simulink model "EMG_Model_Simulink"  (R2019a)
settings: Solver=VariableStepAuto  StartTime=0.0  StopTime=180  RelTol=1e-3
libraries: dsparch4 x2, simulink x1
settings Model: Creator=patri  LastModifiedBy=patri

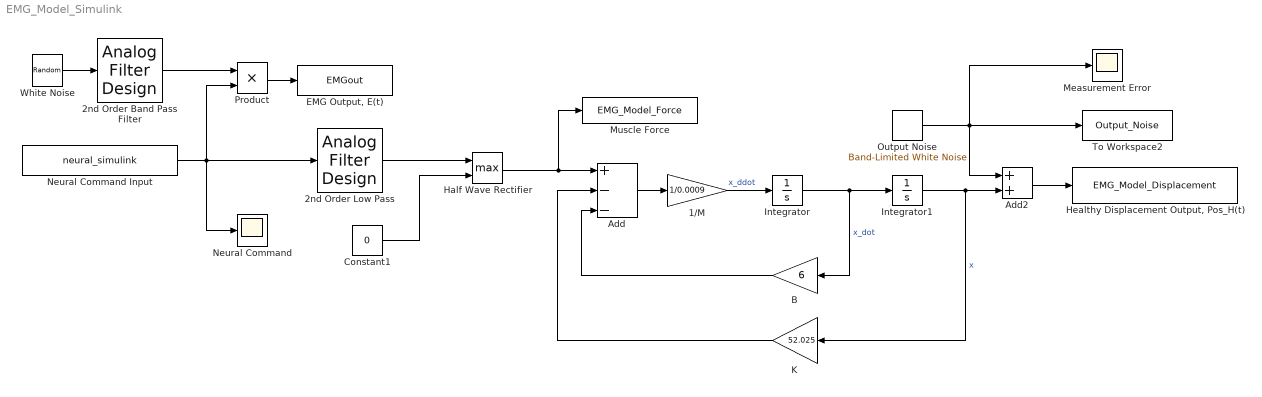
== system EMG_Model_Simulink ==
  1/M : Gain  Gain=1/0.0009
  2nd Order Band Pass Filter : dsparch4/Analog Filter Design  method=Butterworth  filttype=Bandpass  N=2  Wlo=62.83  Whi=3141.59  Rp=2  Rs=40
  2nd Order Low Pass : dsparch4/Analog Filter Design  method=Butterworth  filttype=Lowpass  N=2  Wlo=6.28*2  Whi=80  Rp=2  Rs=40
  Add : Sum  Inputs=+--
  Add2 : Sum
  B : Gain  Gain=6
  Constant1 : Constant  Value=0
  "EMG Output, E(t)" : ToWorkspace  VariableName=EMGout  SampleTime=0.001
  Half Wave Rectifier : MinMax  Function=max  Inputs=2
  "Healthy Displacement Output, Pos_H(t)" : ToWorkspace  VariableName=EMG_Model_Displacement  SampleTime=0.001
  Integrator : Integrator
  Integrator1 : Integrator
  K : Gain  Gain=52.025
  Measurement Error : Scope
  Muscle Force : ToWorkspace  VariableName=EMG_Model_Force  SampleTime=0.001
  Neural Command : Scope
  Neural Command Input : FromWorkspace  VariableName=neural_simulink  SampleTime=0.001
  Output Noise : simulink/Sources/Band-Limited White Noise  Cov=set_output_noise_power  Ts=0.001  seed=22334
  Product : Product
  To Workspace2 : ToWorkspace  VariableName=Output_Noise  SampleTime=0.001
  White Noise : UniformRandomNumber  Minimum=-6.2e-4  Maximum=6.2e-4  SampleTime=0.001
  wires:
  White Noise/1 -> 2nd Order Band Pass Filter/1
  Neural Command Input/1 -> Neural Command/1, 2nd Order Low Pass/1, Product/2
  Add/1 -> 1/M/1
  1/M/1 -> Integrator/1  "x_ddot"
  Integrator/1 -> B/1, Integrator1/1  "x_dot"
  Integrator1/1 -> K/1, Add2/2  "x"
  B/1 -> Add/3
  Half Wave Rectifier/1 -> Add/1, Muscle Force/1
  2nd Order Band Pass Filter/1 -> Product/1
  Product/1 -> "EMG Output, E(t)"/1
  2nd Order Low Pass/1 -> Half Wave Rectifier/1
  Constant1/1 -> Half Wave Rectifier/2
  K/1 -> Add/2
  Output Noise/1 -> Add2/1, To Workspace2/1, Measurement Error/1
  Add2/1 -> "Healthy Displacement Output, Pos_H(t)"/1
